simulink model "unipolar_SPWM"  (R2021a)
settings: Solver=VariableStepAuto  StartTime=0.0  StopTime=10.0  RelTol=1e-3
libraries: spsRMSLib x11, fl_lib x7, spsDiodeLib x5, spsCurrentMeasurementLib x4, spsMosfetLib x4, nesl_utility x4, spsVoltageMeasurementLib x4, spsSeriesRLCBranchLib x3, simulink x2, spsTriangleGeneratorLib x2, spsACVoltageSourceLib x1, spsCurrentVoltageSimscapeInterfaceLib x1
settings Model: Creator=Ahmed  LastModifiedBy=Ahmed

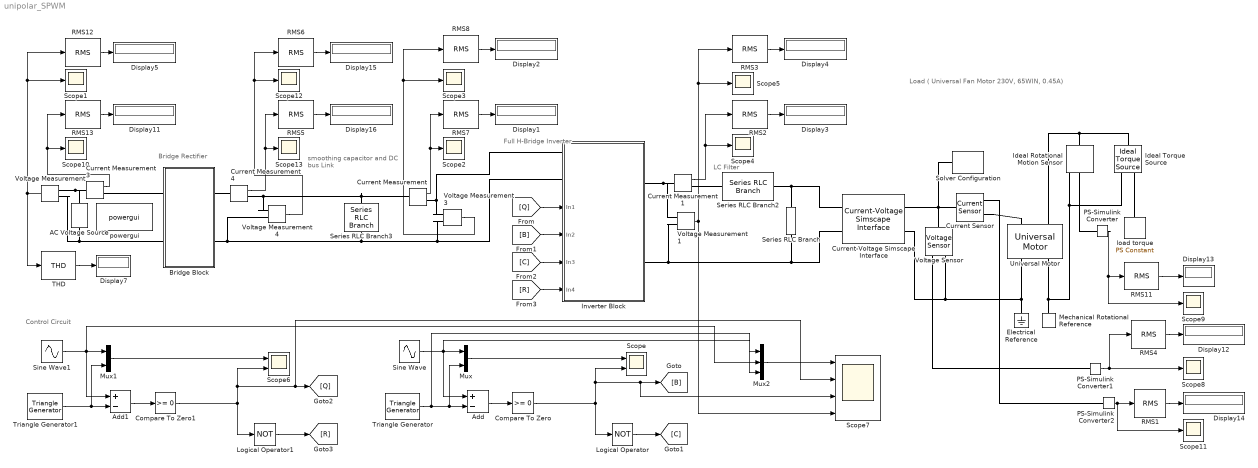
== system unipolar_SPWM ==
  note: Full H-Bridge Inverter
  note: Load ( Universal Fan Motor 230V, 65WIN, 0.45A)
  note: LC Filter
  note: smoothing capacitor
      | and DC bus Link
  note: Control Circuit
  note: Bridge Rectifier
  AC Voltage Source : spsACVoltageSourceLib/AC Voltage Source  Amplitude=220*sqrt(2)  Phase=0  Frequency=50  SampleTime=0  Measurements=None  BusType=swing  Pref=10e3  Qref=0  Qmin=-inf  Qmax=+inf
  Add : Sum  Inputs=+-
  Add1 : Sum  Inputs=+-
  Bridge Block : Subsystem
  Compare To Zero : simulink/Logic and Bit Operations/Compare To Zero  relop=>=  OutDataTypeStr=boolean
  Compare To Zero1 : simulink/Logic and Bit Operations/Compare To Zero  relop=>=  OutDataTypeStr=boolean
  Current Measurement{,1,3..4} (4 alike) : spsCurrentMeasurementLib/Current Measurement  PhasorSimulation=off  OutputType=Complex  PSBequivalent=0
  Current Sensor : fl_lib/Electrical/Electrical Sensors/Current Sensor
  Current-Voltage Simscape Interface : spsCurrentVoltageSimscapeInterfaceLib/Current-Voltage Simscape Interface  DFT=on  FMode=Low pass filter (continuous)  T=1e-6  Ts=50e-6  i0=0  v0=0  Sd=Specialized Power Systems side  Measurements=off
      settings: SourceProductBaseCode=PS
  Display{1..5,7,11..16} (12 alike) : Display
  Electrical Reference : fl_lib/Electrical/Electrical Elements/Electrical Reference
  Ideal Rotational Motion Sensor : fl_lib/Mechanical/Mechanical Sensors/Ideal Rotational Motion Sensor  wrap_angle=simscape.enum.onoff.off  offset=0 rad
  Ideal Torque Source : fl_lib/Mechanical/Mechanical Sources/Ideal Torque Source
  Inverter Block : Subsystem
      settings: PortSchema="{\"entries\":[{\"content\":{\"sides\":[{\"content\":{\"connectorIds\":[\"LConn1\",\"LConn2\",\"In1\",\"In2\",\"In3\",\"In4\"]},\"type\":\"ConnectorPlacement.EquallySpacedRectSide\",\"uuid\":\"1bf4b2d0-4854-4c0e-8872-e91514c85725\"},{\"content\":{\"connectorIds\":[\"RConn1\",\"RConn2\"],\"side\":\"RIGHT\"},\"type\":\"ConnectorPlacement.EquallySpacedRectSide\",\"uuid\":\"cfdf8c94-44a8-440a-96d0-aa9ff41b9350\"},{\"content\":{\"connectorIds\":[],\"side\":\"TOP\"},\"type\":\"ConnectorPlacement.EquallySpacedRectSide\",\"uuid\":\"a545767d-34d0-4732-92d4-780125b27bb8\"}]},\"type\":\"ConnectorPlacement.EquallySpacedConnector\",\"uuid\":\"78f0d0b1-084b-4d4e-b3c7-1214e74f6801\"}],\"packageUris\":[\"http://schema.mathworks.com/mf0/Connector/R2020b\"],\"version\":\"1.0\"}"
  Logical Operator : Logic  Operator=NOT  AllPortsSameDT=off  OutDataTypeStr=boolean
  Logical Operator1 : Logic  Operator=NOT  AllPortsSameDT=off  OutDataTypeStr=boolean
  Mechanical Rotational Reference : fl_lib/Mechanical/Rotational Elements/Mechanical Rotational Reference
  Mux : Mux  Inputs=2
  Mux1 : Mux  Inputs=2
  Mux2 : Mux  Inputs=3
  PS-Simulink Converter : nesl_utility/PS-Simulink Converter  PhysicalDomain=network_engine_domain  SubClassName=ps_output  LeftPortType=input  RightPortType=output  PseudoPeriodic=off  Frequencies=[]  Unit=inherit  AffineConversion=off
      settings: SourceProductBaseCode=PW,SS
  PS-Simulink Converter1 : nesl_utility/PS-Simulink Converter  PhysicalDomain=network_engine_domain  SubClassName=ps_output  LeftPortType=input  RightPortType=output  PseudoPeriodic=off  Frequencies=[]  Unit=inherit  AffineConversion=off
      settings: SourceProductBaseCode=PW,SS
  PS-Simulink Converter2 : nesl_utility/PS-Simulink Converter  PhysicalDomain=network_engine_domain  SubClassName=ps_output  LeftPortType=input  RightPortType=output  PseudoPeriodic=off  Frequencies=[]  Unit=inherit  AffineConversion=off
      settings: SourceProductBaseCode=PW,SS
  RMS{1..8,11..13} (11 alike) : spsRMSLib/RMS  TrueRMS=on  Freq=50  RMSInit=0  Ts=0
  Scope : Scope  NumInputPorts=2
  Scope{1..5,8..13} (11 alike) : Scope
  Scope6 : Scope  NumInputPorts=2
  Scope7 : Scope  NumInputPorts=4
  Series RLC Branch : spsSeriesRLCBranchLib/Series RLC Branch  LConnTagsString=__new0  RConnTagsString=__new0  BranchType=C  Resistance=10  Inductance=100e-6  SetiL0=off  InitialCurrent=0  Capacitance=220e-9  Setx0=off  InitialVoltage=0  Measurements=None
  Series RLC Branch2 : spsSeriesRLCBranchLib/Series RLC Branch  LConnTagsString=__new0  RConnTagsString=__new0  BranchType=L  Resistance=10  Inductance=120e-3  SetiL0=off  InitialCurrent=0  Capacitance=1e-6  Setx0=off  InitialVoltage=0  Measurements=None
  Series RLC Branch3 : spsSeriesRLCBranchLib/Series RLC Branch  LConnTagsString=__new0  RConnTagsString=__new0  BranchType=C  Resistance=10  Inductance=1e-3  SetiL0=off  InitialCurrent=0  Capacitance=220e-6  Setx0=off  InitialVoltage=0  Measurements=None
  Sine Wave : Sin  Frequency=2*pi*50  Phase=pi  SampleTime=0
  Sine Wave1 : Sin  Frequency=2*pi*50  SampleTime=0
  Solver Configuration : nesl_utility/Solver Configuration  PhysicalDomain=network_engine_domain  SubClassName=solver  LeftPortType=input  RightPortType=generic  Tones=[]  Harmonics=[]  SimulateNoise=off  Profile=off  UseLocalSampling=off  EnableSwitchedLinearOptims=on  FrequencyDomain=off  UseCCode=off  RelTol=0.001  AbsTol=1e-06  MinStep=1e-09  ToWorkspace=off  RevertToSquareIcSolve=off  NumHomotopyIterations=100  PhasorMode=off  PhasorModeNumHarmonics=1  DoDC=off  ResidualTolerance=1e-09  UseLocalSolver=off  LocalSolverChoice=NE_BACKWARD_EULER_ADVANCER  LocalSolverSampleTime=0.001  DoFixedCost=off  MaxNonlinIter=3  MaxModeIter=2  ComputeImpulses=off  ImpulseIterations=2  LinearAlgebra=auto  EquationFormulation=NE_TIME_EF  DelaysMemoryBudget=1024  AutomaticFiltering=on  FilteringTimeConstant=0.001  PartitionStorageMethod=AS_NEEDED  PartitionMemoryBudget=1024  PartitionMethod=ROBUST
      settings: SourceProductBaseCode=PW,SS
  THD : spsTHDLib/THD  Freq=50  Ts=0
      settings: SourceProductBaseCode=PS
  Triangle Generator : spsTriangleGeneratorLib/Triangle Generator  Freq=50*101  Phase=0  Ts=0
  Triangle Generator1 : spsTriangleGeneratorLib/Triangle Generator  Freq=50*101  Phase=0  Ts=0
  Universal Motor : ee_lib/Electromechanical/Brushed Motors/Universal Motor  parameterization=4  Ra=132.8 Ohm  Laf=0.1722 s*V/rad/A  w_rated=1300 rpm  P_rated=16 W  V_dc=200 V  T_max=0.39 N*m  P_in=65 W  V_ac=230 V  I_ac=0.45 A  w_ac=50 Hz  Ltot=0.525 H  J=2e-4 kg*m^2  lam=1e-6 N*m/(rad/s)  speed0=0 rpm  resistance_ratio=1  alpha=[.00393, .00393] 1/K  Tmeas=25 degC  thermal_masses=[100, 100] J/K  initial_temperatures=[25, 25] degC
      settings: SourceProductBaseCode=PS  InternalSimscapePortConfiguration="{\"Bottom\":[],\"Left\":[{\"id\":\"p\",\"label\":\"+\",\"type\":\"foundation.electrical.electrical\"},{\"id\":\"R\",\"label\":\"R\",\"type\":\"foundation.mechanical.rotational.rotational\"}],\"Right\":[{\"id\":\"n\",\"label\":\"-\",\"type\":\"foundation.electrical.electrical\"},{\"id\":\"C\",\"label\":\"C\",\"type\":\"foundation.mechanical.rotational.rotational\"}],\"Top\":[]}"
  Voltage Measurement{,1,3..4} (4 alike) : spsVoltageMeasurementLib/Voltage Measurement  PhasorSimulation=off  OutputType=Complex  PSBequivalent=0
  Voltage Sensor : fl_lib/Electrical/Electrical Sensors/Voltage Sensor
  load torque : fl_lib/Physical Signals/Sources/PS Constant  constant=0.1175 N*m
  powergui : spspowerguiLib/powergui  Priority=1  SimulationMode=Discrete  SampleTime=1e-6  frequency=60  Iterations=50  frequencyindice=50  Pbase=100e6  ErrMax=1e-4  UnitsV=kV  UnitsW=MW  buscounter=0  FunctionMessages=off  echomessages=off  EnableUseOfTLC=off  CurrentSourceSwitches=off  DisableSnubberDevices=off  DisableRonSwitches=off  DisableVfSwitches=off  DisplayEquations=off  AutomaticDiscreteSolvers=off  SolverType=Tustin/Backward Euler (TBE)  Interpol=off  ExternalGateDelay=off  methode=off  Ts=100  x0status=blocks  SPID=on  SwTol=0  HookPort=off  NonlinearTolerance=1e-4  nMaxIteration=100  ContinueOnMaxIteration=off  RestoreLinks=warning  ResistiveCurrentMeasurement=off  Frange=[0:2:500]  Ylog=off  Xlog=on  ShowGrid=off  save=off  variable=ZData  structure=0  ZoomFFT=off  StartTime=0.0  cycles=1  DisplayStyle=1  fundamental=60  FreqAxis=off  MaxFrequency=1000  frequencyindicesteady=1  RmsSteady=1  display=off
  wires:
  RMS4/1 -> Display12/1
  Voltage Measurement4/1 -> RMS6/1, Scope12/1
  RMS6/1 -> Display15/1
  RMS5/1 -> Display16/1
  [C] -> Inverter Block/3(In3)
  Sine Wave/1 -> Mux2/1, Add/1, Mux/1
  [B] -> Inverter Block/2(In2)
  [Q] -> Inverter Block/1(In1)
  PS-Simulink Converter2/1 -> RMS1/1, Scope11/1
  RMS8/1 -> Display2/1
  Logical Operator/1 -> [C]
  Triangle Generator/1 -> Mux2/3, Mux/2, Add/2
  PS-Simulink Converter1/1 -> RMS4/1, Scope8/1
  RMS11/1 -> Display13/1
  RMS1/1 -> Display14/1
  RMS7/1 -> Display1/1
  RMS3/1 -> Display4/1
  RMS2/1 -> Display3/1
  Current Measurement/1 -> RMS7/1, Scope2/1
  Add/1 -> Compare To Zero/1
  Current Measurement3/1 -> RMS13/1, Scope10/1
  Current Measurement1/1 -> Scope4/1, RMS2/1
  Voltage Measurement/1 -> RMS12/1, Scope1/1, THD/1
  Current Measurement4/1 -> RMS5/1, Scope13/1
  Voltage Measurement3/1 -> Scope3/1, RMS8/1
  Compare To Zero/1 -> Scope/2, Scope7/3, [B], Logical Operator/1
  RMS12/1 -> Display5/1
  RMS13/1 -> Display11/1
  [R] -> Inverter Block/4(In4)
  Mux/1 -> Scope/1
  THD/1 -> Display7/1
  Voltage Measurement1/1 -> Scope5/1, RMS3/1, Scope7/4
  PS-Simulink Converter/1 -> RMS11/1, Scope9/1
  Mux1/1 -> Scope6/1
  Compare To Zero1/1 -> Scope6/2, Scope7/2, [Q], Logical Operator1/1
  Add1/1 -> Compare To Zero1/1
  Triangle Generator1/1 -> Mux1/2, Add1/2
  Logical Operator1/1 -> [R]
  Sine Wave1/1 -> Mux2/2, Add1/1, Mux1/1
  Mux2/1 -> Scope7/1
  connections:
  Inverter Block/RConn1 -- Current Measurement1/LConn1 -- Voltage Measurement1/LConn1
  Inverter Block/RConn2 -- Current-Voltage Simscape Interface/LConn2 -- Series RLC Branch/RConn1 -- Voltage Measurement1/LConn2
  AC Voltage Source/LConn1 -- Voltage Measurement/LConn2 -- Bridge Block/LConn2
  Ideal Torque Source/RConn2 -- Ideal Rotational Motion Sensor/RConn1 -- Universal Motor/RConn2 -- Mechanical Rotational Reference/LConn1
  Ideal Rotational Motion Sensor/LConn1 -- Universal Motor/LConn2 -- Ideal Torque Source/LConn1
  Inverter Block/LConn2 -- Voltage Measurement3/LConn2 -- Voltage Measurement4/LConn2 -- Bridge Block/RConn2 -- Series RLC Branch3/RConn1
  Current Measurement4/RConn1 -- Series RLC Branch3/LConn1 -- Current Measurement/LConn1 -- Voltage Measurement4/LConn1
  Voltage Sensor/LConn1 -- Current-Voltage Simscape Interface/RConn1 -- Solver Configuration/RConn1 -- Current Sensor/LConn1
  Current-Voltage Simscape Interface/RConn2 -- Voltage Sensor/RConn2 -- Universal Motor/RConn1 -- Electrical Reference/LConn1
  Current Measurement3/LConn1 -- AC Voltage Source/RConn1 -- Voltage Measurement/LConn1
  Current Measurement/RConn1 -- Inverter Block/LConn1 -- Voltage Measurement3/LConn1
  Series RLC Branch2/RConn1 -- Series RLC Branch/LConn1 -- Current-Voltage Simscape Interface/LConn1
  PS-Simulink Converter2/LConn1 -- Current Sensor/RConn1
  Current Sensor/RConn2 -- Universal Motor/LConn1
  Current Measurement1/RConn1 -- Series RLC Branch2/LConn1
  Current Measurement4/LConn1 -- Bridge Block/RConn1
  Voltage Sensor/RConn1 -- PS-Simulink Converter1/LConn1
  load torque/RConn1 -- Ideal Torque Source/RConn1
  Current Measurement3/RConn1 -- Bridge Block/LConn1
  PS-Simulink Converter/LConn1 -- Ideal Rotational Motion Sensor/RConn2

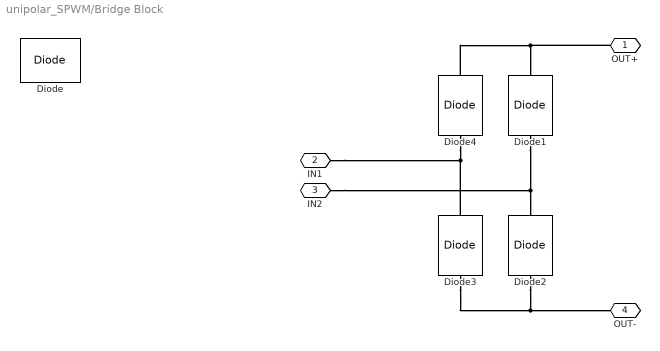
== system unipolar_SPWM/Bridge Block ==
  Diode : spsDiodeLib/Diode  Ron=0.001  Lon=0  Vf=0.8  IC=0  UseSnubber=0  Rs=500  Cs=250e-9  Measurements=on
  Diode{1..4} (4 alike) : spsDiodeLib/Diode  Ron=0.001  Lon=0  Vf=0.7  IC=0  UseSnubber=0  Rs=500  Cs=250e-9  Measurements=off
  OUT+ : PMIOPort  Side=Right
  IN1 : PMIOPort  Port=2  Side=Left
  IN2 : PMIOPort  Port=3  Side=Left
  OUT- : PMIOPort  Port=4  Side=Right
  connections:
  Diode1/LConn1 -- IN2/RConn1 -- Diode2/RConn1
  Diode4/RConn1 -- Diode1/RConn1 -- OUT+/RConn1
  Diode3/RConn1 -- IN1/RConn1 -- Diode4/LConn1
  Diode2/LConn1 -- Diode3/LConn1 -- OUT-/RConn1

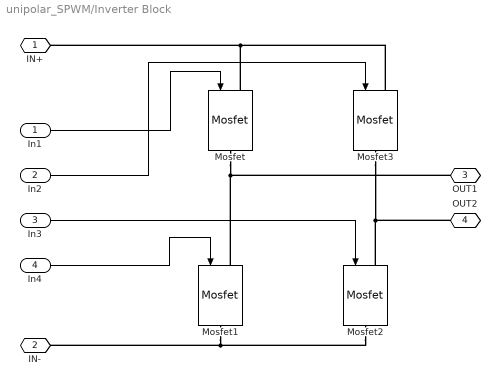
== system unipolar_SPWM/Inverter Block ==
  In1 : Inport
  In2 : Inport  Port=2
  In3 : Inport  Port=3
  In4 : Inport  Port=4
  Mosfet{,1..3} (4 alike) : spsMosfetLib/Mosfet  Ron=0.85  Lon=0  Rd=0.01  Vfd=0.7  IC=0  Rs=470  Cs=10e-9  Measurements=off
  IN+ : PMIOPort  Side=Left
  IN- : PMIOPort  Port=2  Side=Left
  OUT1 : PMIOPort  Port=3  Side=Right
  OUT2 : PMIOPort  Port=4  Side=Right
  wires:
  In1/1 -> Mosfet/1
  In2/1 -> Mosfet3/1
  In3/1 -> Mosfet2/1
  In4/1 -> Mosfet1/1
  connections:
  Mosfet2/LConn1 -- OUT2/RConn1 -- Mosfet3/RConn1
  Mosfet2/RConn1 -- Mosfet1/RConn1 -- IN-/RConn1
  Mosfet/RConn1 -- OUT1/RConn1 -- Mosfet1/LConn1
  Mosfet/LConn1 -- Mosfet3/LConn1 -- IN+/RConn1
